simulink model "s0506_test"  (R2019b)
settings: Solver=ode1  StartTime=0.0  StopTime=25  FixedStep=dt  RelTol=1e-3
values from neighbouring files (symbols this model uses):
  dt = 1e-4    (= 0.0001)    [m0303_init.m]    (also in m0310_init.m = mean(diff(log.time)); m0312_init.m; m0314_init.m = 0.002; m0318_init.m = 0.0002)
  PARAMS =     [s0310_main.mat]
undefined symbols (not defined in the file or in its folder): __PRM__SERIALIZED__DATA__, SubsystemReferenceBlock
libraries: simulink x1
settings Model: Creator=paolo  LastModifiedBy=alessandro
settings DebuggingCC: AlgebraicLoopMsg=none  SFMachineParentedDataDiag=error  ArithmeticOperatorsInVariantConditions=warning
settings SFSimCC: CustomCodeUndefinedFunction=UseInterfaceOnly
settings CodeAppCC: StateflowObjectComments=on

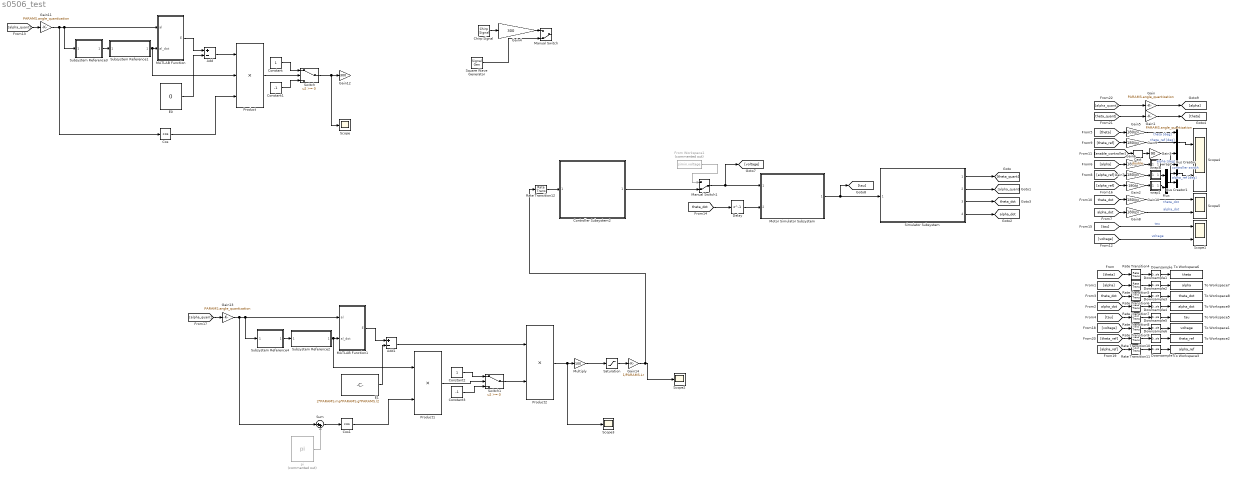
== system s0506_test ==
  Add : Sum  Inputs=+-
  Add1 : Sum  Inputs=+-
  Bus Creator : BusCreator  Inputs=3
  Bus Creator1 : BusCreator  Inputs=3
  Cast : DataTypeConversion  OutDataTypeStr=double
  Chirp Signal : simulink/Sources/Chirp Signal  f1=1  T=50  f2=10
  Constant : Constant
  Constant1 : Constant  Value=-1
  Constant2 : Constant
  Constant3 : Constant  Value=-1
  Controller Subsystem2 : Subsystem  ReferencedSubsystem=s0506_th_ddot_pid
  Cos : Trigonometry  Operator=cos
  Cos1 : Trigonometry  Operator=cos
  Delay : Delay  DelayLength=1  InitialCondition=PARAMS.th_dot_0
  Downsample{,1..7} (8 alike) : DownSample  N=ceil((2e-3)/dt)  RateOptions=Allow multirate processing
  E0 : Constant  Value=0
  E1 : Constant  Value=2*PARAMS.mp*PARAMS.g*PARAMS.l2
  From Workspace1 : FromWorkspace  Commented=on  VariableName=simin.voltage  SampleTime=0
  Gain{,1,11,13} (4 alike) : Gain  Gain=PARAMS.angle_quantization
  Gain{5..10} (6 alike) : Gain  Gain=180/pi
  Gain12 : Gain  Gain=300
  Gain14 : Gain  Gain=1/PARAMS.Lr
  Gain2 : Gain  Gain=-180/pi
  Gain3 : Gain  Gain=90
  Gain4 : Gain  Gain=300
  MATLAB Function : MATLAB Function  TreatAsAtomicUnit=on
  MATLAB Function1 : MATLAB Function  TreatAsAtomicUnit=on
  Manual Switch : ManualSwitch  CurrentSetting=0
  Manual Switch1 : ManualSwitch  CurrentSetting=0
  Motor Simulator Subsystem : Subsystem  ReferencedSubsystem=s0303_motor_simulator  omega_0=PARAMS.th_dot_0  i_0=0
  Multiply : Gain  Gain=100
  Mux : Mux  Inputs=2
  Product : Product  Inputs=3
  Product1 : Product
  Product2 : Product
  Rate Transition{4..11} (8 alike) : RateTransition  OutPortSampleTime=dt
  Rate Transition12 : RateTransition  OutPortSampleTime=dt_control
  Saturation : Saturate  UpperLimit=200  LowerLimit=-200
  Scope : Scope
  Scope1 : Scope  NumInputPorts=2
  Scope2 : Scope
  Scope3 : Scope
  Scope4 : Scope  NumInputPorts=2
  Scope5 : Scope  NumInputPorts=2
  Simulator Subsystem : Subsystem  ReferencedSubsystem=s0405_mechanical_simulator  th_0=PARAMS.th_0  al_0=PARAMS.al_0  th_dot_0=PARAMS.th_dot_0  al_dot_0=PARAMS.al_dot_0
  Square Wave Generator : SignalGenerator  WaveForm=square  Amplitude=120
  Subsystem Reference1 : Subsystem  BlockKeywords=__PRM__SERIALIZED__DATA__:SubsystemReferenceBlock  ReferencedSubsystem=Filtered_Derivative  num=num_der_filter  den=den_der_filter
  Subsystem Reference2 : Subsystem  BlockKeywords=__PRM__SERIALIZED__DATA__:SubsystemReferenceBlock  ReferencedSubsystem=Filtered_Derivative  num=num_der_filter  den=den_der_filter
  Subsystem Reference3 : Subsystem  BlockKeywords=__PRM__SERIALIZED__DATA__:SubsystemReferenceBlock  ReferencedSubsystem=Polynomial_Filter
  Subsystem Reference4 : Subsystem  BlockKeywords=__PRM__SERIALIZED__DATA__:SubsystemReferenceBlock  ReferencedSubsystem=Polynomial_Filter
  Sum : Sum  Inputs=|++
  Switch : Switch
  Switch1 : Switch
  To Workspace1 : ToWorkspace  VariableName=voltage  SaveFormat=Timeseries  SampleTime=-1
  To Workspace2 : ToWorkspace  VariableName=theta_ref  SaveFormat=Timeseries  SampleTime=-1
  To Workspace3 : ToWorkspace  VariableName=alpha_ref  SaveFormat=Timeseries  SampleTime=-1
  To Workspace5 : ToWorkspace  VariableName=tau  SaveFormat=Timeseries  SampleTime=-1
  To Workspace6 : ToWorkspace  VariableName=theta  SaveFormat=Timeseries  SampleTime=-1
  To Workspace7 : ToWorkspace  VariableName=alpha  SaveFormat=Timeseries  SampleTime=-1
  To Workspace8 : ToWorkspace  VariableName=theta_dot  SaveFormat=Timeseries  SampleTime=-1
  To Workspace9 : ToWorkspace  VariableName=alpha_dot  SaveFormat=Timeseries  SampleTime=-1
  pi : Constant  Commented=on  Value=pi
  wrap1 : MATLAB Function  TreatAsAtomicUnit=on
  wrap2 : MATLAB Function  TreatAsAtomicUnit=on
  wrap3 : MATLAB Function  TreatAsAtomicUnit=on
  tag scope: alpha_dot=global, theta_dot=global
  wires:
  Simulator Subsystem/1 -> [theta_quant]
  Simulator Subsystem/2 -> [alpha_quant]
  Simulator Subsystem/4 -> [alpha_dot]
  Simulator Subsystem/3 -> [theta_dot]
  Motor Simulator Subsystem/1 -> Simulator Subsystem/1, [tau]
  Bus Creator/1 -> Scope4/1
  [alpha_ref] -> Gain7/1
  [theta] -> Gain5/1
  [alpha] -> Gain6/1
  Gain8/1 -> Scope5/2  "alpha_dot"
  Bus Creator1/1 -> Scope4/2
  [theta_dot] -> Gain10/1
  [alpha_dot] -> Gain8/1
  Gain10/1 -> Scope5/1  "theta_dot"
  [theta_ref] -> Gain9/1
  [theta_dot] -> Delay/1
  [voltage] -> Scope1/2  "voltage"
  [tau] -> Scope1/1  "tau"
  Delay/1 -> Motor Simulator Subsystem/2
  [theta] -> Rate Transition4/1
  [alpha] -> Rate Transition5/1
  [theta_dot] -> Rate Transition6/1
  [alpha_dot] -> Rate Transition7/1
  [tau] -> Rate Transition8/1
  [voltage] -> Rate Transition9/1
  [theta_ref] -> Rate Transition10/1
  [alpha_ref] -> Rate Transition11/1
  Downsample7/1 -> To Workspace3/1
  Downsample6/1 -> To Workspace2/1
  Downsample5/1 -> To Workspace1/1
  Downsample4/1 -> To Workspace5/1
  Downsample3/1 -> To Workspace9/1
  Downsample2/1 -> To Workspace8/1
  Downsample1/1 -> To Workspace7/1
  Downsample/1 -> To Workspace6/1
  Rate Transition4/1 -> Downsample/1
  Rate Transition5/1 -> Downsample1/1
  Rate Transition6/1 -> Downsample2/1
  Rate Transition7/1 -> Downsample3/1
  Rate Transition8/1 -> Downsample4/1
  Rate Transition9/1 -> Downsample5/1
  Rate Transition10/1 -> Downsample6/1
  Rate Transition11/1 -> Downsample7/1
  Gain9/1 -> Bus Creator/2  "theta_ref [deg]"
  wrap2/1(y) -> Bus Creator1/1  "alpha [deg]"
  Gain6/1 -> wrap2/1(u)
  Gain7/1 -> wrap3/1(u)
  Gain5/1 -> Bus Creator/1  "theta [deg]"
  [alpha_quant] -> Gain/1
  Gain/1 -> [alpha]
  Gain1/1 -> [theta]
  [theta_quant] -> Gain1/1
  Rate Transition12/1 -> Controller Subsystem2/1
  wrap3/1(y) -> Mux/1
  Mux/1 -> Bus Creator1/2  "alpha_ref [deg]"
  Gain2/1 -> wrap1/1(u)
  [alpha_ref] -> Gain2/1
  wrap1/1(y) -> Mux/2
  [enable_controller] -> Cast/1
  Gain3/1 -> Bus Creator1/3, Bus Creator/3  "controller switch"
  Cast/1 -> Gain3/1
  Manual Switch1/1 -> [voltage], Motor Simulator Subsystem/1
  From Workspace1/1 -> Manual Switch1/1
  Controller Subsystem2/1 -> Manual Switch1/2
  Chirp Signal/1 -> Gain4/1
  Gain4/1 -> Manual Switch/1
  Square Wave Generator/1 -> Manual Switch/2
  Gain11/1 -> Cos/1, MATLAB Function/1(al), Subsystem Reference3/1
  [alpha_quant] -> Gain11/1
  Subsystem Reference3/1 -> Subsystem Reference1/1
  Subsystem Reference1/1 -> Product/2, MATLAB Function/2(al_dot)
  MATLAB Function/1(E) -> Add/1
  E0/1 -> Add/2
  Add/1 -> Product/1
  Cos/1 -> Product/3
  Product/1 -> Switch/2
  Constant/1 -> Switch/1
  Constant1/1 -> Switch/3
  Switch/1 -> Scope/1, Gain12/1
  Constant3/1 -> Switch1/3
  Constant2/1 -> Switch1/1
  Product1/1 -> Switch1/2
  Cos1/1 -> Product1/2
  E1/1 -> Add1/2
  MATLAB Function1/1(E) -> Add1/1
  Subsystem Reference2/1 -> Product1/1, MATLAB Function1/2(al_dot)
  Subsystem Reference4/1 -> Subsystem Reference2/1
  [alpha_quant] -> Gain13/1
  Gain13/1 -> Sum/1, Subsystem Reference4/1, MATLAB Function1/1(al)
  Switch1/1 -> Product2/2
  Add1/1 -> Product2/1
  Product2/1 -> Scope3/1, Multiply/1
  Multiply/1 -> Saturation/1
  Saturation/1 -> Gain14/1
  Gain14/1 -> Rate Transition12/1, Scope2/1
  pi/1 -> Sum/2
  Sum/1 -> Cos1/1

== matlab function s0506_test/wrap2 ==
  data: u input; y output
function y = wrap(u)
stop_condition = false;
y = u;
while ~stop_condition
    if y > 270
        y = y - 360;
    elseif y < -270
        y = y + 360;
    else
        stop_condition = true;
    end
end

== matlab function s0506_test/wrap3 ==
  data: u input; y output
function y = wrap(u)
stop_condition = false;
y = u;
while ~stop_condition
    if y > 270
        y = y - 360;
    elseif y < -270
        y = y + 360;
    else
        stop_condition = true;
    end
end

== matlab function s0506_test/wrap1 ==
  data: u input; y output
function y = wrap(u)
stop_condition = false;
y = u;
while ~stop_condition
    if y > 270
        y = y - 360;
    elseif y < -270
        y = y + 360;
    else
        stop_condition = true;
    end
end

== matlab function s0506_test/MATLAB Function ==
  data: al input; E output; al_dot input; PARAMS parameter
function E = energy(al, al_dot, PARAMS)
    
    J=1/12*PARAMS.Lp^2*PARAMS.mp + PARAMS.l2^2*PARAMS.mp;
    
    
    
E = 1/2*J*al_dot^2+PARAMS.mp*PARAMS.g*PARAMS.l2*(cos(al+pi)-1);

== matlab function s0506_test/MATLAB Function1 ==
  data: al input; E output; al_dot input; PARAMS parameter
function E = energy(al, al_dot, PARAMS)
    
    J=1/12*PARAMS.Lp^2*PARAMS.mp + PARAMS.l2^2*PARAMS.mp;
    
    
    
E = 1/2*J*al_dot^2+PARAMS.mp*PARAMS.g*PARAMS.l2*(1-cos(al));
